simulink model "tutorial13_dc_motor"  (R2025a)
settings: Solver=VariableStepAuto  StartTime=0.0  StopTime=1.5  RelTol=1e-3
settings Model: Creator=xing2  LastModifiedBy=xing2

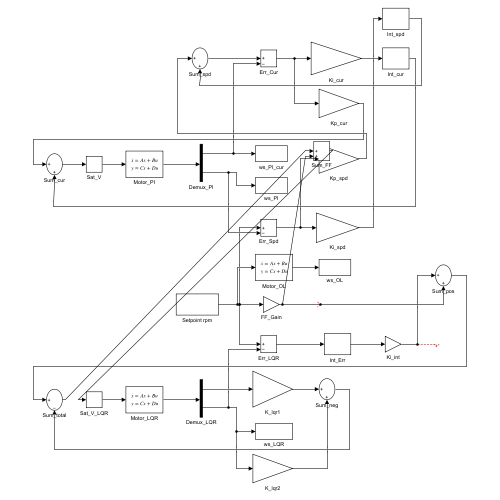
[thumbnail: Simulink's stored preview of the top-level diagram]
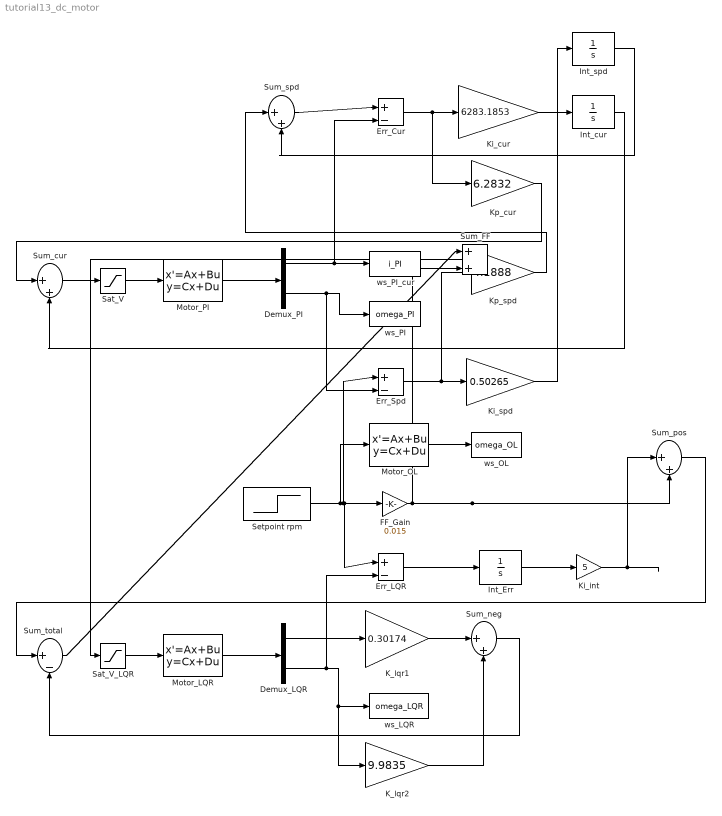
== system tutorial13_dc_motor ==
  Demux_LQR : Demux  Outputs=2
  Demux_PI : Demux  Outputs=2
  Err_Cur : Sum  Inputs=|+-
  Err_LQR : Sum  Inputs=|+-
  Err_Spd : Sum  Inputs=|+-
  FF_Gain : Gain  Gain=0.015
  Int_Err : Integrator
  Int_cur : Integrator
  Int_spd : Integrator
  K_lqr1 : Gain  Gain=0.30174
  K_lqr2 : Gain  Gain=9.9835
  Ki_cur : Gain  Gain=6283.1853
  Ki_int : Gain  Gain=5
  Ki_spd : Gain  Gain=0.50265
  Kp_cur : Gain  Gain=6.2832
  Kp_spd : Gain  Gain=4.1888
  Motor_LQR : StateSpace  A=[-1000 -7.5;30 -0.02]  B=[500;0]  C=eye(2)  D=zeros(2,1)  InitialCondition=[0; 0]
  Motor_OL : StateSpace  A=[-1000 -7.5;30 -0.02]  B=[500;0]  C=[0 1]  D=0  InitialCondition=[0; 0]
  Motor_PI : StateSpace  A=[-1000 -7.5;30 -0.02]  B=[500;0]  C=eye(2)  D=zeros(2,1)  InitialCondition=[0; 0]
  Sat_V : Saturate  UpperLimit=12  LowerLimit=-12
  Sat_V_LQR : Saturate  UpperLimit=12  LowerLimit=-12
  Setpoint rpm : Step  Time=0.01  After=100  SampleTime=0
  Sum_FF : Sum  Inputs=|++
  Sum_cur : Sum  Inputs=|++
  Sum_neg : Sum  Inputs=|++
  Sum_pos : Sum  Inputs=|++
  Sum_spd : Sum  Inputs=|++
  Sum_total : Sum  Inputs=|+-
  ws_LQR : ToWorkspace  VariableName=omega_LQR  SaveFormat=Timeseries  SampleTime=-1
  ws_OL : ToWorkspace  VariableName=omega_OL  SaveFormat=Timeseries  SampleTime=-1
  ws_PI : ToWorkspace  VariableName=omega_PI  SaveFormat=Timeseries  SampleTime=-1
  ws_PI_cur : ToWorkspace  VariableName=i_PI  SaveFormat=Timeseries  SampleTime=-1
  wires:
  Sum_cur/1 -> Sat_V/1
  Motor_LQR/1 -> Demux_LQR/1
  Ki_spd/1 -> Int_spd/1
  Demux_PI/1 -> Err_Cur/2, ws_PI_cur/1
  Sat_V_LQR/1 -> Motor_LQR/1
  Err_Spd/1 -> Kp_spd/1, Ki_spd/1
  Demux_LQR/1 -> K_lqr1/1
  Sat_V/1 -> Motor_PI/1
  Motor_PI/1 -> Demux_PI/1
  Ki_cur/1 -> Int_cur/1
  Sum_spd/1 -> Err_Cur/1
  Ki_int/1 -> Sum_pos/1
  Demux_PI/2 -> Err_Spd/2, ws_PI/1
  Setpoint rpm/1 -> Err_LQR/1, FF_Gain/1, Err_Spd/1, Motor_OL/1
  Demux_LQR/2 -> K_lqr2/1, ws_LQR/1, Err_LQR/2
  Err_Cur/1 -> Kp_cur/1, Ki_cur/1
  Motor_OL/1 -> ws_OL/1
  FF_Gain/1 -> Sum_pos/2, Sum_FF/2
  Err_LQR/1 -> Int_Err/1
  K_lqr1/1 -> Sum_neg/1
  K_lqr2/1 -> Sum_neg/2
  Kp_cur/1 -> Sum_cur/1
  Kp_spd/1 -> Sum_spd/1
  Int_Err/1 -> Ki_int/1
  Sum_neg/1 -> Sum_total/2
  Int_spd/1 -> Sum_spd/2
  Int_cur/1 -> Sum_cur/2
  Sum_pos/1 -> Sum_total/1
  Sum_total/1 -> Sum_FF/1
  Sum_FF/1 -> Sat_V_LQR/1
